simulink model "DYN_02x"  (R2021a)
settings: Solver=FixedStepAuto  StartTime=0.0  StopTime=10  FixedStep=0.01  RelTol=1e-3
(part 1 of 14)
settings Model: Creator=TMP  LastModifiedBy=TMP
settings SolverCC: AlgebraicLoopSolver=TrustRegion
settings DebuggingCC: SFMachineParentedDataDiag=warning  ArithmeticOperatorsInVariantConditions=warning
settings SFSimCC: CustomCodeUndefinedFunction=UseInterfaceOnly

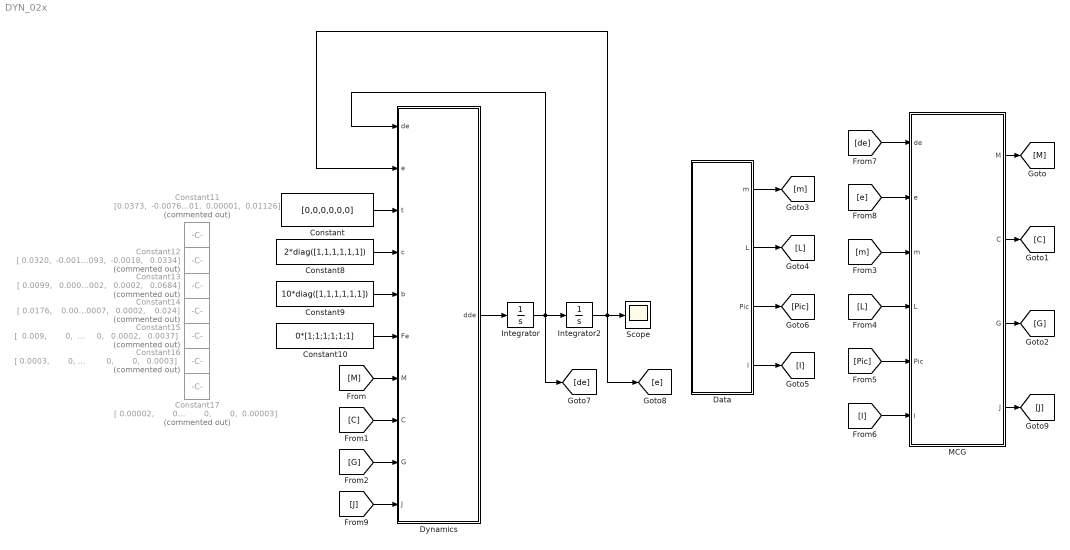
== system DYN_02x ==
  Constant : Constant  Value=[0,0,0,0,0,0]
  Constant10 : Constant  Value=0*[1;1;1;1;1;1]
  Constant11 : Constant  Commented=on  Value=|
      | [0.0373,  -0.0076,   0.1064;
      |        0.1127,   0.0065,   0.0648;
      |        0.0447,   0.0125,  -0.0554;
      |        0.0006,   0.0052,   0.1068;
      |             0,   0.0062,   0.0195;
      |      -0.00001,  0.00001,  0.01126]
  Constant12 : Constant  Commented=on  Value=|
      | [ 0.0320,  -0.0017,   0.0093;
      |       -0.0017,   0.0364,  -0.0018;
      |        0.0093,  -0.0018,   0.0334]
  Constant13 : Constant  Commented=on  Value=|
      | [ 0.0099,   0.0008,  -0.0002;
      |        0.0008,   0.0646,   0.0002;
      |       -0.0002,   0.0002,   0.0684]
  Constant14 : Constant  Commented=on  Value=|
      | [ 0.0176,    0.001,   0.0007;
      |         0.001,   0.0195,   0.0002;
      |        0.0007,   0.0002,    0.024]
  Constant15 : Constant  Commented=on  Value=|
      | [  0.009,        0,        0;
      |             0,   0.0081,   0.0002;
      |             0,   0.0002,   0.0037]
  Constant16 : Constant  Commented=on  Value=|
      | [ 0.0003,        0,        0;
      |             0,   0.0002,        0;
      |             0,        0,   0.0003]
  Constant17 : Constant  Commented=on  Value=|
      | [ 0.00002,        0,        0;
      |              0,  0.00002,        0;
      |              0,        0,  0.00003]
  Constant8 : Constant  Value=2*diag([1,1,1,1,1,1])
  Constant9 : Constant  Value=10*diag([1,1,1,1,1,1])
  Data : MATLAB Function  TreatAsAtomicUnit=on
  Dynamics : MATLAB Function  TreatAsAtomicUnit=on
  Integrator : Integrator  InitialCondition=[0;0;0;0;0;0]
  Integrator2 : Integrator  InitialCondition=[0;0;0;0;0;0]
  MCG : MATLAB Function  TreatAsAtomicUnit=on
  Scope : Scope
  wires:
  Integrator2/1 -> [e], Scope/1, Dynamics/2(e)
  Dynamics/1(dde) -> Integrator/1
  Integrator/1 -> [de], Integrator2/1, Dynamics/1(de)
  Constant8/1 -> Dynamics/4(c)
  Constant9/1 -> Dynamics/5(b)
  Constant10/1 -> Dynamics/6(Fe)
  MCG/1(M) -> [M]
  MCG/2(C) -> [C]
  MCG/3(G) -> [G]
  [M] -> Dynamics/7(M)
  [C] -> Dynamics/8(C)
  [G] -> Dynamics/9(G)
  Data/1(m) -> [m]
  Data/2(L) -> [L]
  Data/3(Pic) -> [Pic]
  Data/4(I) -> [I]
  [L] -> MCG/4(L)
  [Pic] -> MCG/5(Pic)
  [I] -> MCG/6(I)
  Constant/1 -> Dynamics/3(t)
  [m] -> MCG/3(m)
  [de] -> MCG/1(de)
  [e] -> MCG/2(e)
  MCG/4(J) -> [J]
  [J] -> Dynamics/10(J)

== matlab function DYN_02x/Dynamics ==
  data: de input; e input; t input; c input; b input; Fe input; M input; dde output; C input; G input; J input
function dde = DYN_6DOF(de,e,t,c,b,Fe,M,C,G,J)
%%
e1 = e(1); e2 = e(2); e3 = e(3);
e4 = e(4); e5 = e(5); e6 = e(6);
de1 = de(1); de2 = de(2); de3 = de(3);
de4 = de(4); de5 = de(5); de6 = de(6);


%%
de = [de1;de2;de3;de4;de5;de6];
F = c*sign(de) + b*de + J'*Fe ;
dde = M\(t-C*de-G-F);
